simulink model "Simu_Model_vs_Logs"  (R2018b)
settings: Solver=FixedStepAuto  StartTime=0.0  StopTime=60  FixedStep=.00005  RelTol=1e-3
undefined symbols (not defined in the file or in its folder): sim2mat
libraries: simulink x1
Description:
  | Compare model of a Pravalux DC motor with real values recorded:
  | Current and Speed were previously recorded with a shirp and with a large steps input voltage stimulus.
  | 
  | Same input are injected to the motor model and its output validated against real record.
  | 
  | The input file with record can be selected (from file block).
settings Model: Creator=Lubin Kerhuel - Romain Delpoux  LastModifiedBy=Lubin Kerhuel

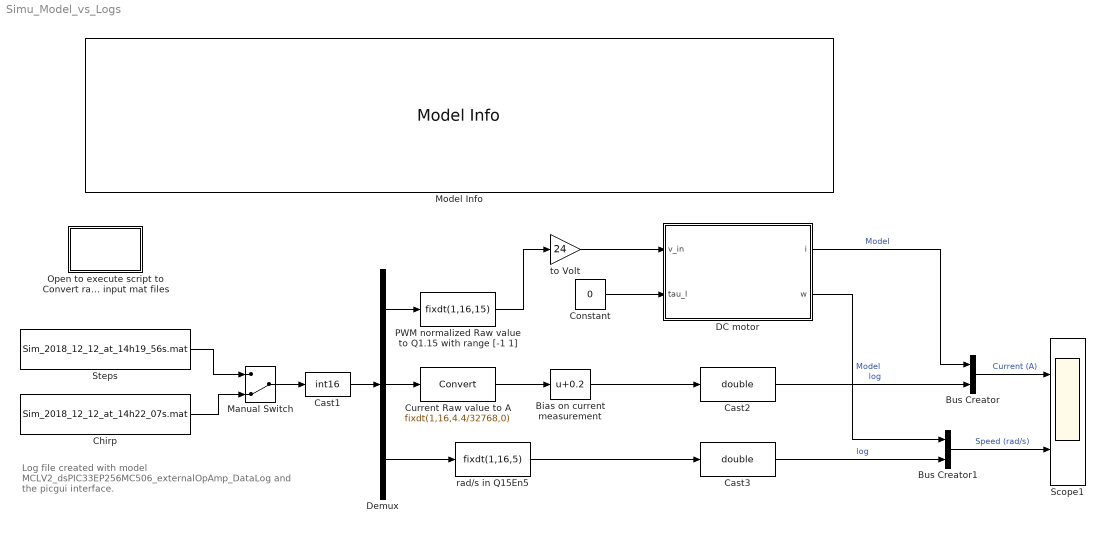
== system Simu_Model_vs_Logs ==
  note: Log file created with model
      | MCLV2_dsPIC33EP256MC506_externalOpAmp_DataLog
      | and the picgui interface.
  Bias on current measurement : Bias  Bias=0.2  SaturateOnIntegerOverflow=on
  Bus Creator : BusCreator  Inputs=2
  Bus Creator1 : BusCreator  Inputs=2
  Cast1 : DataTypeConversion  OutDataTypeStr=int16
  Cast2 : DataTypeConversion  OutDataTypeStr=double
  Cast3 : DataTypeConversion  OutDataTypeStr=double
  Chirp : FromFile  FileName=Sim_2018_12_12_at_14h22_07s.mat  SampleTime=.00005
  Constant : Constant  Value=0
  Current Raw value to A : DataTypeConversion  OutDataTypeStr=fixdt(1,16,4.4/32768,0)  ConvertRealWorld=Stored Integer (SI)
  DC motor : Subsystem  mask(Motor PRAVALUX MPM4-0002){R=1.22, L=0.0027, Kphi=0.061, J=0.22e-3, F=.0001, C0=-0.032, mod=0.25*0}
      mask prompts: R "Resistance (R) in Ohms"; L "Inductance (L) in H"; Kphi "Back EMF (Kphi) in V/rad/s"; J "J in kgm²"; F "F in N/rad/s"; mod "BEMF modulation (default: 0.25, 0 for off)"
      mask help:
      | Continuous time Model for PRAVALUX MPM4 DC motor
      | Caracteristics: 24V DC, 90W, 5.2A, 3000RPM
      |
      | It is a 2nd order model made of two intertwinned system:
      | one 1st order electrical system and one 1st order mechanical system.
      |
      | Modulation on the BEMF can be added to fit with motor current ripple measured
      |
      | Look under mask (Ctrl-U) to see the model
      mask DialogControl Container11 Prompt: Motor
      mask DialogControl Container3 Prompt: Electrical Parameters
      mask DialogControl Container3_copy Prompt: Mechanical Parameters
      mask DialogControl Container14 Prompt: BEMF modulation
      mask Display:
      | color('green');
      | image('MotorPravalux.png');
      | %port_label('input',1,'DC');
      | %port_label('output',1,'BEMF');
  Demux : Demux  Outputs=3
  Manual Switch : ManualSwitch  CurrentSetting=0
  Model Info : simulink/Model-Wide Utilities/Model Info  Frame=off  DisplayStringWithTags=|  HorizontalTextAlignment=Center  LeftAlignmentValue=0.5
      | %<ModelName> - %<LastModificationDate>
      | %<Creator>
      | 
      | %<Description>
  Open to execute script to Convert raw input mat files : Subsystem  LoadFcn=sim2mat();
      settings: OpenFcn=sim2mat();
  PWM normalized Raw value to Q1.15 with range [-1 1] : DataTypeConversion  OutDataTypeStr=fixdt(1,16,15)  ConvertRealWorld=Stored Integer (SI)
  Scope1 : Scope  NumInputPorts=2
  Steps : FromFile  FileName=Sim_2018_12_12_at_14h19_56s.mat  SampleTime=.00005
  rad/s in Q15En5 : DataTypeConversion  OutDataTypeStr=fixdt(1,16,5)  ConvertRealWorld=Stored Integer (SI)
  to Volt : Gain  Gain=24  OutDataTypeStr=double
  wires:
  Manual Switch/1 -> Cast1/1
  Demux/1 -> PWM normalized Raw value to Q1.15 with range [-1 1]/1
  Demux/2 -> Current Raw value to A/1
  Demux/3 -> rad/s in Q15En5/1
  PWM normalized Raw value to Q1.15 with range [-1 1]/1 -> to Volt/1
  Current Raw value to A/1 -> Bias on current measurement/1
  rad/s in Q15En5/1 -> Cast3/1
  Cast1/1 -> Demux/1
  to Volt/1 -> DC motor/1(v_in)
  Steps/1 -> Manual Switch/1
  Chirp/1 -> Manual Switch/2
  DC motor/2(w) -> Bus Creator1/1  "Model"
  DC motor/1(i) -> Bus Creator/1  "Model"
  Bus Creator/1 -> Scope1/1  "Current (A)"
  Bus Creator1/1 -> Scope1/2  "Speed (rad/s)"
  Constant/1 -> DC motor/2(tau_l)
  Bias on current measurement/1 -> Cast2/1
  Cast2/1 -> Bus Creator/2  "log"
  Cast3/1 -> Bus Creator1/2  "log"

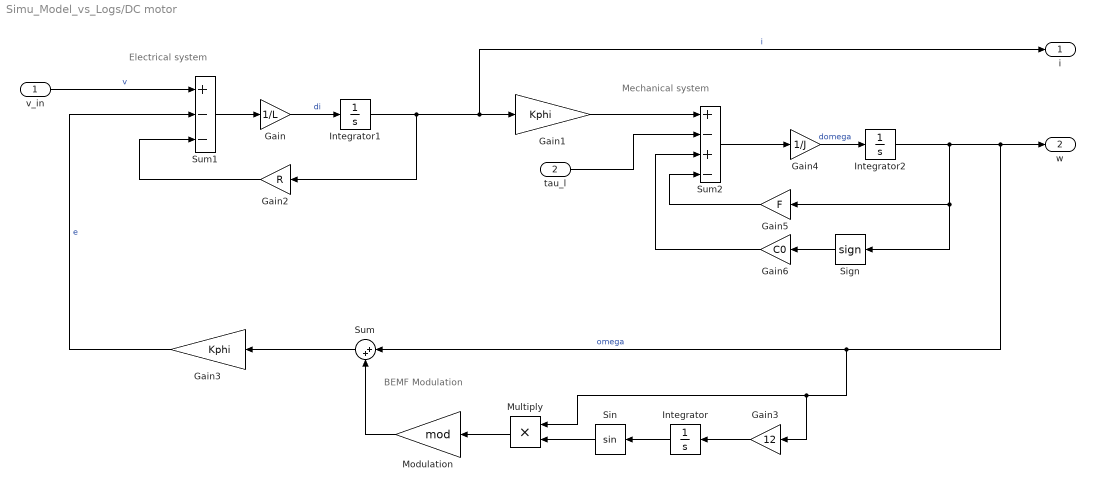
== system Simu_Model_vs_Logs/DC motor ==
  note: BEMF Modulation
  note: Mechanical system
  note: Electrical system
  v_in : Inport  SampleTime=0
  tau_l : Inport  Port=2
  Gain : Gain  Gain=1/L
  Gain1 : Gain  Gain=Kphi
  Gain2 : Gain  Gain=R
  Gain3 : Gain  Gain=12
  "Gain3  " : Gain  Gain=Kphi
  Gain4 : Gain  Gain=1/J
  Gain5 : Gain  Gain=F
  Gain6 : Gain  Gain=C0
  Integrator : Integrator  WrapState=on
  Integrator1 : Integrator
  Integrator2 : Integrator
  Modulation : Gain  Gain=mod
  Multiply : Product
  Sign : Signum
  Sin : Trigonometry
  Sum : Sum  Inputs=|++
  Sum1 : Sum  Inputs=+--
  Sum2 : Sum  Inputs=+-+-
  i : Outport
  w : Outport  Port=2
  wires:
  Sin/1 -> Multiply/2
  Sum/1 -> "Gain3  "/1
  Modulation/1 -> Sum/2
  Multiply/1 -> Modulation/1
  Integrator/1 -> Sin/1
  Gain3/1 -> Integrator/1
  Sum1/1 -> Gain/1
  Gain/1 -> Integrator1/1  "di"
  Integrator1/1 -> Gain2/1, i/1, Gain1/1  "i"
  v_in/1 -> Sum1/1  "v"
  Gain2/1 -> Sum1/3
  "Gain3  "/1 -> Sum1/2  "e"
  tau_l/1 -> Sum2/2
  Gain6/1 -> Sum2/3
  Sign/1 -> Gain6/1
  Integrator2/1 -> w/1, Sum/1, Gain3/1, Multiply/1, Sign/1, Gain5/1  "omega"
  Gain5/1 -> Sum2/4
  Sum2/1 -> Gain4/1
  Gain4/1 -> Integrator2/1  "domega"
  Gain1/1 -> Sum2/1

== system Simu_Model_vs_Logs/Open to execute script to Convert raw input mat files ==
